simulink model "dcmotorss1"  (R2025b)
settings: Solver=VariableStepAuto  StartTime=0.0  StopTime=10.0  RelTol=1e-3
undefined symbols (not defined in the file): b, J, K, L, R, T_ref, W_ref
libraries: slpidlib x1
settings Model: Creator=adity  LastModifiedBy=adity

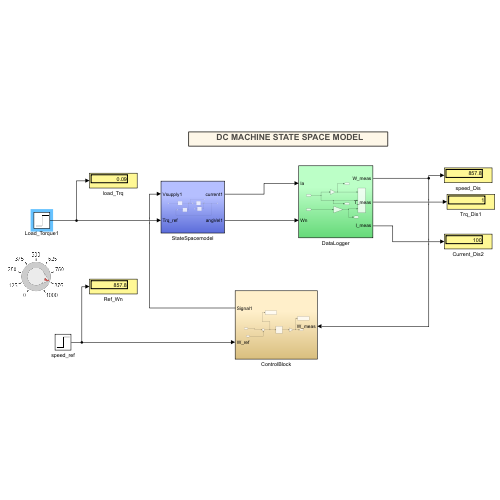
[thumbnail: Simulink's stored preview of the top-level diagram]
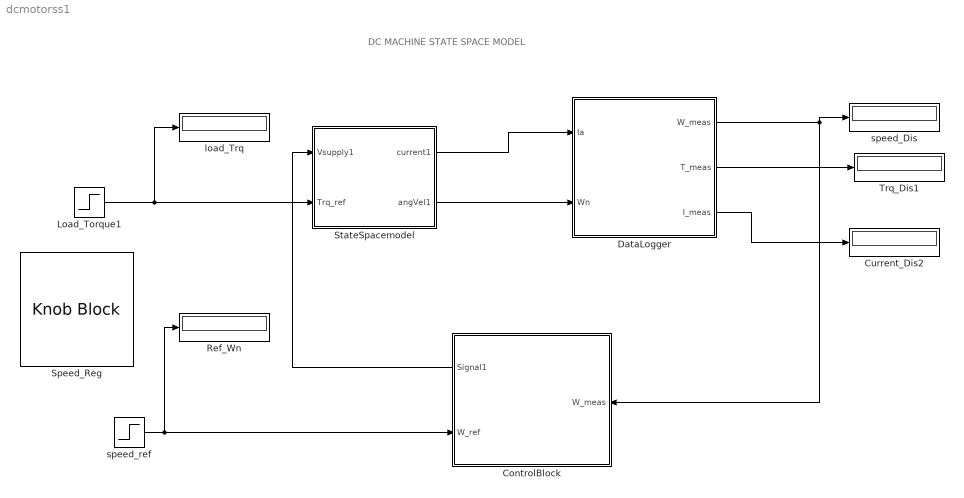
== system dcmotorss1 ==
  note: DC MACHINE STATE SPACE MODEL
  ControlBlock : Subsystem
      settings: PortSchema="{\"entries\":[{\"content\":{\"sides\":[{\"content\":{\"connectorIds\":[\"Out1\",\"In1\"]},\"type\":\"ConnectorPlacement.EquallySpacedRectSide\",\"uuid\":\"e873ae36-8892-4051-8497-27d8e059c7b4\"},{\"content\":{\"connectorIds\":[\"In2\"],\"side\":\"RIGHT\"},\"type\":\"ConnectorPlacement.EquallySpacedRectSide\",\"uuid\":\"1081217f-3a68-4f59-94a1-2fdbd8c85e76\"},{\"content\":{\"side\":\"TOP\"},\"type\":\"ConnectorPlacement.EquallySpacedRectSide\",\"uuid\":\"bf2c7dc1-5542-4291-8e07-a6fe84c89847\"}]},\"type\":\"ConnectorPlacement.EquallySpacedConnector\",\"uuid\":\"d2293d51-49ef-4c2e-bb75-5f57d6512c86\"}],\"packageUris\":[\"http://schema.mathworks.com/mf0/Connector/R2020b\"],\"version\":\"1.0\"}"
  Current_Dis2 : Display
  DataLogger : Subsystem
  Load_Torque1 : Step  After=T_ref  SampleTime=0
  Ref_Wn : Display
  Speed_Reg : KnobBlock  LabelPosition=Hide  ScaleMax=1000
  StateSpacemodel : Subsystem
  Trq_Dis1 : Display
  load_Trq : Display
  speed_Dis : Display
  speed_ref : Step  After=W_ref  SampleTime=0
  wires:
  DataLogger/1(W_meas) -> ControlBlock/2(W_meas), speed_Dis/1
  ControlBlock/1(Signal1) -> StateSpacemodel/1(Vsupply1)
  StateSpacemodel/1(current1) -> DataLogger/1(Ia)
  StateSpacemodel/2(angVel1) -> DataLogger/2(Wn)
  Load_Torque1/1 -> load_Trq/1, StateSpacemodel/2(Trq_ref)
  speed_ref/1 -> ControlBlock/1(W_ref), Ref_Wn/1
  DataLogger/2(T_meas) -> Trq_Dis1/1
  DataLogger/3(I_meas) -> Current_Dis2/1

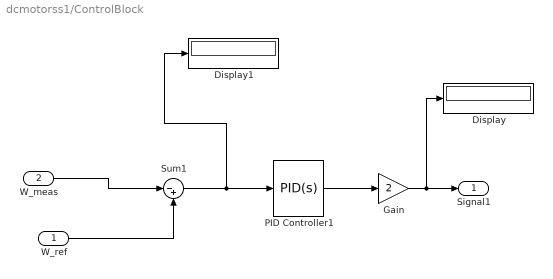
== system dcmotorss1/ControlBlock ==
  W_ref : Inport
  W_meas : Inport  Port=2
  Display : Display
  Display1 : Display
  Gain : Gain  Gain=2
  PID Controller1 : slpidlib/PID Controller  Controller=PID  Form=Parallel  TimeDomain=Continuous-time  UseExternalTs=off  SampleTime=-1  IntegratorMethod=Forward Euler  FilterMethod=Forward Euler  ControllerParametersSource=internal  P=1  I=0.9  UseKiTs=off  D=0.05  UseExternalDerivativeSource=off  N=100  UseFilter=on  TunerSelectOption=Transfer Function Based (PID Tuner App)  InitialConditionSource=internal  InitialConditionForIntegrator=0  InitialConditionForFilter=0  DifferentiatorICPrevScaledInput=0  ExternalReset=none  TrackingMode=off  Kt=1  LimitOutput=off  SatLimitsSource=internal  UpperSaturationLimit=inf  LowerSaturationLimit=-inf  LinearizeAsGain=on  AntiWindupMode=none  Kb=1  LimitIntegrator=off  UpperIntegratorSaturationLimit=inf  LowerIntegratorSaturationLimit=-inf  POutMin=[]  POutMax=[]  IOutMin=[]  IOutMax=[]  DOutMin=[]  DOutMax=[]  NOutMin=[]  NOutMax=[]  SumOutMin=[]  SumOutMax=[]  SaturationOutMin=[]  SaturationOutMax=[]  PParamMin=[]  PParamMax=[]  IParamMin=[]  IParamMax=[]  DParamMin=[]  DParamMax=[]  NParamMin=[]  NParamMax=[]  KbParamMin=[]  KbParamMax=[]  KtParamMin=[]  KtParamMax=[]  KbOutMin=[]  KbOutMax=[]  KtOutMin=[]  KtOutMax=[]  IntegratorOutMin=[]  IntegratorOutMax=[]  FilterOutMin=[]  FilterOutMax=[]  SumI1OutMin=[]  SumI1OutMax=[]  SumI2OutMin=[]  SumI2OutMax=[]  SumI3OutMin=[]  SumI3OutMax=[]  SumI4OutMin=[]  SumI4OutMax=[]  SumDOutMin=[]  SumDOutMax=[]  DifferentiatorOutMin=[]  DifferentiatorOutMax=[]  FilterDiffOutCoefMin=[]  FilterDiffOutCoefMax=[]  ReciprocalOutMin=[]  ReciprocalOutMax=[]  SumDenOutMin=[]  SumDenOutMax=[]  SumNumOutMin=[]  SumNumOutMax=[]  DivideOutMin=[]  DivideOutMax=[]  UdiffTsProdOutMin=[]  UdiffTsProdOutMax=[]  NTsProdOutMin=[]  NTsProdOutMax=[]  UintegralTsProdOutMin=[]  UintegralTsProdOutMax=[]  UngainTsProdOutMin=[]  UngainTsProdOutMax=[]  ClampingZeroOutDataTypeStr=Inherit: Inherit via back propagation  ClampingZeroOutMin=[]  ClampingZeroOutMax=[]  FilterDenConstantOutDataTypeStr=Inherit: Inherit via back propagation  FilterDenConstantOutMin=[]  FilterDenConstantOutMax=[]  PCopyOutDataTypeStr=Inherit: Inherit via back propagation  PCopyOutMin=[]  PCopyOutMax=[]  NCopyOutDataTypeStr=Inherit: Inherit via back propagation  NCopyOutMin=[]  NCopyOutMax=[]  IntegratorContinuousStateAttributes=''  IntegratorStateMustResolveToSignalObject=off  IntegratorRTWStateStorageClass=Auto  FilterContinuousStateAttributes=''  FilterStateMustResolveToSignalObject=off  FilterRTWStateStorageClass=Auto  ParallelPVariant=InternalParameters  IdealPVariant=Disabled  IVariant=InternalParameters  DVariant=InternalParameters  IntegratorVariant=Continuous  SatVariant=Disabled  AWVariant=Passthrough  PCopyVariant=Disabled  TRVariant=Disabled  FdbkBlocksVariant=Forward  IdealPFdbkVariant=Disabled  SatFdbkVariant=Disabled  DerivativeFilterVariant=ContFilter  NVariant=InternalParameters  NCopyVariant=Disabled  FilterICVariant=InternalICsFilter  IntegratorICVariant=InternalICs  ExternalResetVariant=Disabled  TRSumVariant=Passthrough  SumFdbkVariant=Disabled  SumVariant=Sum_PID  TsampFilterVariant=InternalTs  TsampNgainVariant=Passthrough  TsampIntegralVariant=Disabled_SignalSpec  ExternalSaturationOutDataTypeStr=Inherit: Same as second input  DerivativeSourceVariant=ErrorSignal  PreIntVariant=InternalPreInt
  Sum1 : Sum  Inputs=|-+
  Signal1 : Outport
  wires:
  Sum1/1 -> Display1/1, PID Controller1/1
  W_meas/1 -> Sum1/1
  PID Controller1/1 -> Gain/1
  W_ref/1 -> Sum1/2
  Gain/1 -> Display/1, Signal1/1

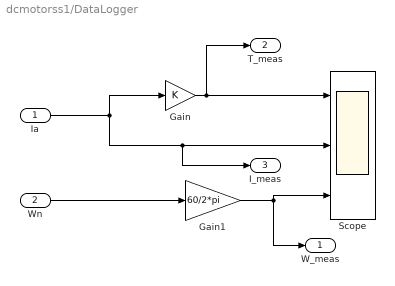
== system dcmotorss1/DataLogger ==
  Ia : Inport
  Wn : Inport  Port=2
  Gain : Gain  Gain=K
  Gain1 : Gain  Gain=60/2*pi
  Scope : Scope  NumInputPorts=3
      settings: ActiveDisplayYMinimum=-1851.8596746326257  ActiveDisplayYMaximum=3301.7336749953711
  W_meas : Outport
  T_meas : Outport  Port=2
  I_meas : Outport  Port=3
  wires:
  Wn/1 -> Gain1/1
  Ia/1 -> Gain/1, I_meas/1, Scope/2
  Gain1/1 -> W_meas/1, Scope/3
  Gain/1 -> Scope/1, T_meas/1

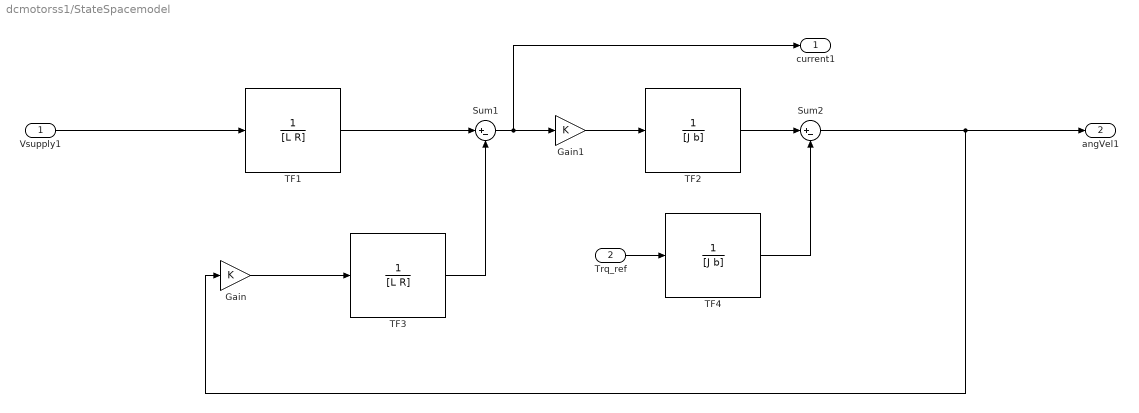
== system dcmotorss1/StateSpacemodel ==
  Vsupply1 : Inport
  Trq_ref : Inport  Port=2
  Gain : Gain  Gain=K
  Gain1 : Gain  Gain=K
  Sum1 : Sum  Inputs=|+-
  Sum2 : Sum  Inputs=|+-
  TF1 : TransferFcn  Numerator=1  Denominator=[L R]
  TF2 : TransferFcn  Numerator=1  Denominator=[J b]
  TF3 : TransferFcn  Numerator=1  Denominator=[L R]
  TF4 : TransferFcn  Numerator=1  Denominator=[J b]
  current1 : Outport
  angVel1 : Outport  Port=2
  wires:
  Gain/1 -> TF3/1
  TF1/1 -> Sum1/1
  TF3/1 -> Sum1/2
  Sum1/1 -> Gain1/1, current1/1
  Gain1/1 -> TF2/1
  TF2/1 -> Sum2/1
  TF4/1 -> Sum2/2
  Sum2/1 -> angVel1/1, Gain/1
  Trq_ref/1 -> TF4/1
  Vsupply1/1 -> TF1/1
